simulink model "homework1_solar"  (R2016a)
settings: Solver=ode1  StartTime=0.0  StopTime=43200  FixedStep=0.1  RelTol=1e-3
undefined symbols (not defined in the file or in its folder): a, eta, i_max
settings Model: Creator=chris.barlow  LastModifiedBy=chris.barlow

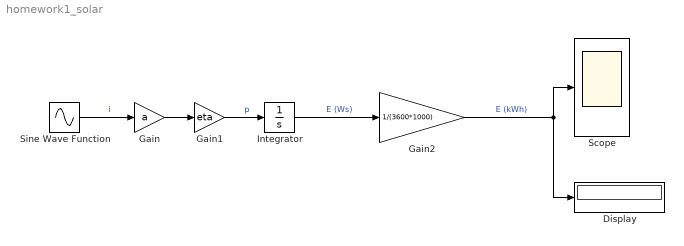
== system homework1_solar ==
  Display : Display
  Gain : Gain  Gain=a
  Gain1 : Gain  Gain=eta
  Gain2 : Gain  Gain=1/(3600*1000)
  Integrator : Integrator
  Scope : Scope
  Sine Wave Function : Sin  Amplitude=i_max  Frequency=pi/(12*3600)  SampleTime=0
  wires:
  Sine Wave Function/1 -> Gain/1  "i"
  Gain/1 -> Gain1/1
  Gain1/1 -> Integrator/1  "p"
  Integrator/1 -> Gain2/1  "E (Ws)"
  Gain2/1 -> Display/1, Scope/1  "E (kWh)"
